simulink library "sm_boom_lift_crawler_lib_actuators"  (R2026a)
settings: Solver=ode23t
undefined symbols (not defined in the file): actuators, BasketR, cylinders, Extend, Jib, LevelM, LevelS, Lift, lines, OutFL, OutFR, OutRL, OutRR, Tilt, TrackL, TrackR, Turret, valves
libraries: SimscapeFluids_lib x92, fl_lib x67, sm_boom_lift_crawler_lib x24, nesl_utility x13, Custom_Valves x2
(part 1 of 5)
Description:
  | Boom Lift Crawler Hydraulics (Library)
  | 
  | Copyright 2020-2026 The MathWorks, Inc.
settings Model: Creator=smiller  LastModifiedBy=smiller

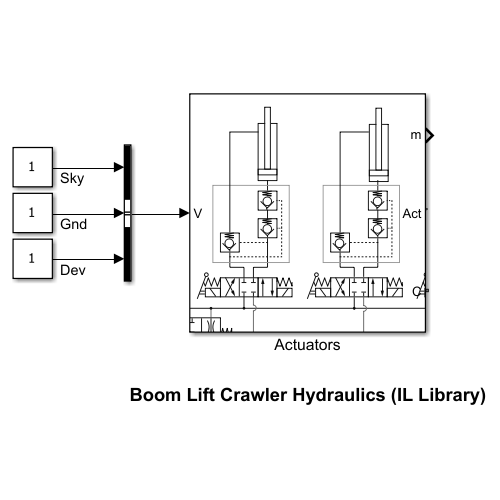
[thumbnail: Simulink's stored preview of the top-level diagram]
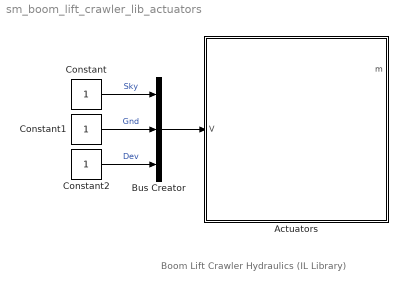
== system sm_boom_lift_crawler_lib_actuators ==
  note: Boom Lift Crawler Hydraulics (IL Library)
  Actuators : Subsystem  VariantControl=Actuators_CVs
      mask Display: image('sh001_trim_2act.svg');
  Bus Creator : BusCreator  Inputs=3
  Constant : Constant
  Constant1 : Constant
  Constant2 : Constant
  wires:
  Constant/1 -> Bus Creator/1  "Sky"
  Constant1/1 -> Bus Creator/2  "Gnd"
  Constant2/1 -> Bus Creator/3  "Dev"
  Bus Creator/1 -> Actuators/1(V)

== system sm_boom_lift_crawler_lib_actuators/Actuators ==
  In Bus Element : Inport  PortName=V  Element=Sky
  In Bus Element1 : Inport  PortName=V  Element=Gnd
  In Bus Element2 : Inport  PortName=V  Element=Dev
  Deviator Valves : Subsystem
      mask Display: image('sh002.svg')
  Ground Manifold : Subsystem
      mask Display: image('sh004.svg')
  Hydraulic Power Unit : Subsystem
      mask Display: image('sh003.svg')
  Sky Manifold : Subsystem
      mask Display: image('sh005.svg')
  Subsystem : Subsystem
  Act : PMIOPort  Side=Right
  C : PMIOPort  Port=2  Side=Right
  m : Outport
  wires:
  In Bus Element/1 -> Sky Manifold/1(Sky)
  In Bus Element2/1 -> Deviator Valves/1(Dev)
  In Bus Element1/1 -> Ground Manifold/1(Gnd)
  [G] -> Subsystem/2(G)
  [S] -> Subsystem/1(S)
  Subsystem/1(H) -> m/1  "Hydr"
  Ground Manifold/1(m) -> [G]
  Sky Manifold/1(m) -> [S]
  connections:
  Ground Manifold/RConn1 -- Sky Manifold/RConn1 -- Act/RConn1
  Sky Manifold/LConn2 -- Deviator Valves/RConn1
  Deviator Valves/RConn3 -- Ground Manifold/LConn3
  Deviator Valves/RConn2 -- Ground Manifold/LConn2
  Sky Manifold/LConn1 -- Ground Manifold/LConn1 -- Hydraulic Power Unit/LConn1 -- C/RConn1
  Deviator Valves/LConn1 -- Hydraulic Power Unit/LConn2
  Deviator Valves/LConn2 -- Hydraulic Power Unit/LConn3

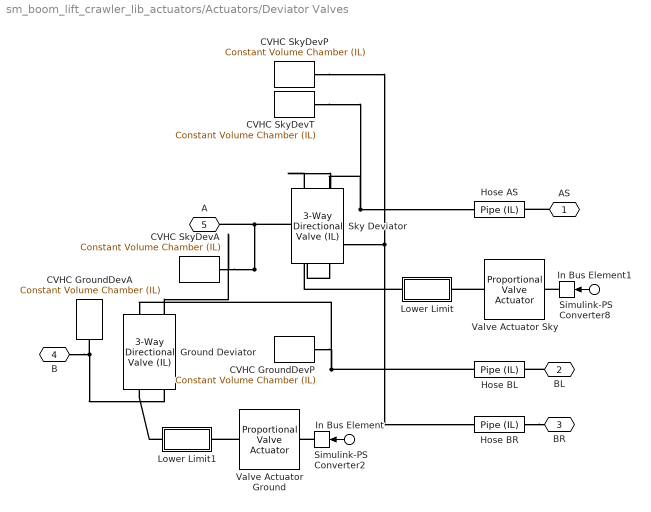
== system sm_boom_lift_crawler_lib_actuators/Actuators/Deviator Valves ==
  In Bus Element : Inport  PortName=Dev  Element=g
  In Bus Element1 : Inport  PortName=Dev  Element=s
  CVHC GroundDevA : fl_lib/Isothermal Liquid/Elements/Constant Volume Chamber (IL)  volume=1e-4 m^3  p_I_specify=off  p_I_priority=High  p_I=0 + 101325 Pa  p_I_nominal_specify=off  p_I_nominal_value=1  p_I_nominal_unit=Pa
  CVHC GroundDevP : fl_lib/Isothermal Liquid/Elements/Constant Volume Chamber (IL)  volume=1e-4 m^3  p_I_specify=off  p_I_priority=High  p_I=0 + 101325 Pa  p_I_nominal_specify=off  p_I_nominal_value=1  p_I_nominal_unit=Pa
  CVHC SkyDevA : fl_lib/Isothermal Liquid/Elements/Constant Volume Chamber (IL)  volume=1e-4 m^3  p_I_specify=off  p_I_priority=High  p_I=0 + 101325 Pa  p_I_nominal_specify=off  p_I_nominal_value=1  p_I_nominal_unit=Pa
  CVHC SkyDevP : fl_lib/Isothermal Liquid/Elements/Constant Volume Chamber (IL)  volume=1e-4 m^3  p_I_specify=off  p_I_priority=High  p_I=0 + 101325 Pa  p_I_nominal_specify=off  p_I_nominal_value=1  p_I_nominal_unit=Pa
  CVHC SkyDevT : fl_lib/Isothermal Liquid/Elements/Constant Volume Chamber (IL)  volume=1e-4 m^3  p_I_specify=off  p_I_priority=High  p_I=0 + 101325 Pa  p_I_nominal_specify=off  p_I_nominal_value=1  p_I_nominal_unit=Pa
  Ground Deviator : SimscapeFluids_lib/Isothermal Liquid/Valves & Orifices/Directional Control Valves/3-Way Directional Valve (IL)  open_orifices_pos=fluids.isothermal_liquid.valves_orifices.directional_control_valves.enum.DirectionalValveOpenOrifices3Way.PA  open_orifices_neg=fluids.isothermal_liquid.valves_orifices.directional_control_valves.enum.DirectionalValveOpenOrifices3Way.AT  area_spec=fluids.isothermal_liquid.valves_orifices.directional_control_valves.enum.directional_valve_area_spec.identical  valve_spec=fluids.isothermal_liquid.valves_orifices.directional_control_valves.enum.directional_valve_spec.linear  del_S_max=(valves.control.l.max) - 1550.0031*(valves.control.l.max)/(lines.ground.main.s.p)*(1e-12) in  area_max=lines.ground.main.s.p in^2  del_S_TLU=([-.002, 0, .002, .005, .015]) - (-0.002) m  valve_area_TLU=[1e-09, 2.0352e-07, 4.0736e-05, .00011438, .00034356] m^2  del_S_vol_flow_TLU=([-.002, 0, .002, .005, .015]) - (-0.002) m  p_diff_TLU=[-10000000, -5000000, -2000000, 2000000, 5000000, 10000000] Pa  vol_flow_TLU=[-1e-07, -7.0711e-08, -4.4721e-08, 4.4721e-08, 7.0711e-08, 1e-07; -2.0352e-05, -1.4391e-05, -9.1017e-06, 9.1017e-06, 1.4391e-05, 2.0352e-05; -.0040736, -.0028805, -.0018218, .0018218, .0028805, .0040736; -.011438, -.0080879, -.0051152, .0051152, .0080879, .011438; -.034356, -.024293, -.015364, .015364, .024293, .034356] m^3/s  area=inf m^2  area_leak=1e-12 m^2  Cd=0.7  Re_c=150  smoothing_factor=0.01  pressure_recovery=false  S_max_PA=-(0) + 0.0254*(valves.control.l.max) m  del_S_max_PA=0.005 m  area_max_PA=0.5e-4 m^2  del_S_TLU_PA=([-.002, 0, .002, .005, .015]) - (-0.002) m  valve_area_TLU_PA=[1e-09, 2.0352e-07, 4.0736e-05, .00011438, .00034356] m^2  del_S_vol_flow_TLU_PA=([-.002, 0, .002, .005, .015]) - (-0.002) m  p_diff_TLU_PA=[-10000000, -5000000, -2000000, 2000000, 5000000, 10000000] Pa  vol_flow_TLU_PA=[-1e-07, -7.0711e-08, -4.4721e-08, 4.4721e-08, 7.0711e-08, 1e-07; -2.0352e-05, -1.4391e-05, -9.1017e-06, 9.1017e-06, 1.4391e-05, 2.0352e-05; -.0040736, -.0028805, -.0018218, .0018218, .0028805, .0040736; -.011438, -.0080879, -.0051152, .0051152, .0080879, .011438; -.034356, -.024293, -.015364, .015364, .024293, .034356] m^3/s  S_max_AT=(0) - 0.0254*(valves.control.l.max) m  del_S_max_AT=0.005 m  area_max_AT=0.5e-4 m^2  del_S_TLU_AT=([-.002, 0, .002, .005, .015]) - (-0.002) m  valve_area_TLU_AT=[1e-09, 2.0352e-07, 4.0736e-05, .00011438, .00034356] m^2  del_S_vol_flow_TLU_AT=([-.002, 0, .002, .005, .015]) - (-0.002) m  p_diff_TLU_AT=[-10000000, -5000000, -2000000, 2000000, 5000000, 10000000] Pa  vol_flow_TLU_AT=[-1e-07, -7.0711e-08, -4.4721e-08, 4.4721e-08, 7.0711e-08, 1e-07; -2.0352e-05, -1.4391e-05, -9.1017e-06, 9.1017e-06, 1.4391e-05, 2.0352e-05; -.0040736, -.0028805, -.0018218, .0018218, .0028805, .0040736; -.011438, -.0080879, -.0051152, .0051152, .0080879, .011438; -.034356, -.024293, -.015364, .015364, .024293, .034356] m^3/s  S_max_PT=2.5e-3 m  del_S_max_PT=0.005 m  area_max_PT=1e-4 m^2  del_S_TLU_PT=[0, .002, .004, .007, .017] m  valve_area_TLU_PT=[1e-09, 2.0352e-07, 4.0736e-05, .00011438, .00034356] m^2  del_S_vol_flow_TLU_PT=[0, .002, .004, .007, .017] m  p_diff_TLU_PT=[.3, .5, .7] MPa  vol_flow_TLU_PT=1e-3 * [1.7e-05, 2e-05, 2.6e-05; .0035, .0045, .0053; .7, .9, 1.06; 1.96, 2.5, 3; 6, 7.7, 9.13] m^3/s
  Hose AS : SimscapeFluids_lib/Isothermal Liquid/Pipes & Fittings/Pipe (IL)  dynamic_compressibility=true  inertia=false  num_segments=1  pipe_length=lines.ground.main.l ft  cross_section_geometry=fluids.isothermal_liquid.pipes_fittings.enum.cross_section_geometry.circular  pipe_diameter=lines.ground.main.d.p in  pipe_inner_diameter=0.05 m  pipe_outer_diameter=0.1 m  pipe_width=0.1 m  pipe_height=0.1 m  pipe_major_axis=0.1 m  pipe_minor_axis=0.05 m  pipe_side=0.1 m  pipe_angle=30 deg  pipe_area=1e-4 m^2  Dh=1.12e-2 m  elevation_spec=foundation.enum.constant_variable.constant  elevation_gain=0 m  gravity_spec=foundation.enum.constant_variable.constant  g=9.81 m/s^2  pressure_loss_spec=fluids.isothermal_liquid.pipes_fittings.enum.pressure_loss_spec.haaland  mdot_nominal=[.1, 1] kg/s  p_diff_nominal=[.001, .01] MPa  mdot_threshold=1e-6 kg/s  local_pressure_loss_spec=fluids.isothermal_liquid.pipes_fittings.enum.local_loss_spec.aggregate_length  length_add=lines.ground.main.lr ft  loss_coefficient=0.1  roughness_spec=fluids.isothermal_liquid.pipes_fittings.enum.roughness_spec.custom  roughness=15e-6 m  Re_friction_TLU=[400, 1000, 1500, 3000, 4000, 6000, 10000, 20000, 40000, 60000, 100000, 100000000]  friction_factor_TLU=[.264, .112, .071, .0417, .0387, .0268, .025, .0232, .0226, .022, .0214, .0214]  Re_lam=2000  Re_tur=4000  shape_factor=64  pipe_wall_spec=fluids.isothermal_liquid.pipes_fittings.enum.wall_spec.rigid  vol_expansion_spec=fluids.isothermal_liquid.pipes_fittings.enum.vol_expansion_spec.area  area_pressure_gain=1e-6 m^2/MPa  static_pressure_TLU=[.1, 1] MPa  area_pressure_gain_TLU=[1e-05, 1.1e-05] m^2  material_behavior_spec=fluids.isothermal_liquid.pipes_fittings.enum.PipeMaterialBehavior.Linear  diameter_pressure_gain=2e-12 m/Pa  wall_thickness=0.05 m  elastic_modulus=69 GPa  stress_TLU=[276, 310] MPa  strain_TLU=[.004, .02]  stress_assert_action=simscape.enum.assert.action.none  stress_max=400 MPa  poisson_ratio=0.33  wall_time_constant=0.01 s  p0=lines.ground.main.p0 + 14.6959 psi  mdot0=0 kg/s
  Hose BL : SimscapeFluids_lib/Isothermal Liquid/Pipes & Fittings/Pipe (IL)  dynamic_compressibility=true  inertia=false  num_segments=1  pipe_length=lines.ground.main.l ft  cross_section_geometry=fluids.isothermal_liquid.pipes_fittings.enum.cross_section_geometry.circular  pipe_diameter=lines.ground.main.d.p in  pipe_inner_diameter=0.05 m  pipe_outer_diameter=0.1 m  pipe_width=0.1 m  pipe_height=0.1 m  pipe_major_axis=0.1 m  pipe_minor_axis=0.05 m  pipe_side=0.1 m  pipe_angle=30 deg  pipe_area=1e-4 m^2  Dh=1.12e-2 m  elevation_spec=foundation.enum.constant_variable.constant  elevation_gain=0 m  gravity_spec=foundation.enum.constant_variable.constant  g=9.81 m/s^2  pressure_loss_spec=fluids.isothermal_liquid.pipes_fittings.enum.pressure_loss_spec.haaland  mdot_nominal=[.1, 1] kg/s  p_diff_nominal=[.001, .01] MPa  mdot_threshold=1e-6 kg/s  local_pressure_loss_spec=fluids.isothermal_liquid.pipes_fittings.enum.local_loss_spec.aggregate_length  length_add=lines.ground.main.lr ft  loss_coefficient=0.1  roughness_spec=fluids.isothermal_liquid.pipes_fittings.enum.roughness_spec.custom  roughness=15e-6 m  Re_friction_TLU=[400, 1000, 1500, 3000, 4000, 6000, 10000, 20000, 40000, 60000, 100000, 100000000]  friction_factor_TLU=[.264, .112, .071, .0417, .0387, .0268, .025, .0232, .0226, .022, .0214, .0214]  Re_lam=2000  Re_tur=4000  shape_factor=64  pipe_wall_spec=fluids.isothermal_liquid.pipes_fittings.enum.wall_spec.rigid  vol_expansion_spec=fluids.isothermal_liquid.pipes_fittings.enum.vol_expansion_spec.area  area_pressure_gain=1e-6 m^2/MPa  static_pressure_TLU=[.1, 1] MPa  area_pressure_gain_TLU=[1e-05, 1.1e-05] m^2  material_behavior_spec=fluids.isothermal_liquid.pipes_fittings.enum.PipeMaterialBehavior.Linear  diameter_pressure_gain=2e-12 m/Pa  wall_thickness=0.05 m  elastic_modulus=69 GPa  stress_TLU=[276, 310] MPa  strain_TLU=[.004, .02]  stress_assert_action=simscape.enum.assert.action.none  stress_max=400 MPa  poisson_ratio=0.33  wall_time_constant=0.01 s  p0=lines.ground.main.p0 + 14.6959 psi  mdot0=0 kg/s
  Hose BR : SimscapeFluids_lib/Isothermal Liquid/Pipes & Fittings/Pipe (IL)  dynamic_compressibility=true  inertia=false  num_segments=1  pipe_length=lines.ground.main.l ft  cross_section_geometry=fluids.isothermal_liquid.pipes_fittings.enum.cross_section_geometry.circular  pipe_diameter=lines.ground.main.d.p in  pipe_inner_diameter=0.05 m  pipe_outer_diameter=0.1 m  pipe_width=0.1 m  pipe_height=0.1 m  pipe_major_axis=0.1 m  pipe_minor_axis=0.05 m  pipe_side=0.1 m  pipe_angle=30 deg  pipe_area=1e-4 m^2  Dh=1.12e-2 m  elevation_spec=foundation.enum.constant_variable.constant  elevation_gain=0 m  gravity_spec=foundation.enum.constant_variable.constant  g=9.81 m/s^2  pressure_loss_spec=fluids.isothermal_liquid.pipes_fittings.enum.pressure_loss_spec.haaland  mdot_nominal=[.1, 1] kg/s  p_diff_nominal=[.001, .01] MPa  mdot_threshold=1e-6 kg/s  local_pressure_loss_spec=fluids.isothermal_liquid.pipes_fittings.enum.local_loss_spec.aggregate_length  length_add=lines.ground.main.lr ft  loss_coefficient=0.1  roughness_spec=fluids.isothermal_liquid.pipes_fittings.enum.roughness_spec.custom  roughness=15e-6 m  Re_friction_TLU=[400, 1000, 1500, 3000, 4000, 6000, 10000, 20000, 40000, 60000, 100000, 100000000]  friction_factor_TLU=[.264, .112, .071, .0417, .0387, .0268, .025, .0232, .0226, .022, .0214, .0214]  Re_lam=2000  Re_tur=4000  shape_factor=64  pipe_wall_spec=fluids.isothermal_liquid.pipes_fittings.enum.wall_spec.rigid  vol_expansion_spec=fluids.isothermal_liquid.pipes_fittings.enum.vol_expansion_spec.area  area_pressure_gain=1e-6 m^2/MPa  static_pressure_TLU=[.1, 1] MPa  area_pressure_gain_TLU=[1e-05, 1.1e-05] m^2  material_behavior_spec=fluids.isothermal_liquid.pipes_fittings.enum.PipeMaterialBehavior.Linear  diameter_pressure_gain=2e-12 m/Pa  wall_thickness=0.05 m  elastic_modulus=69 GPa  stress_TLU=[276, 310] MPa  strain_TLU=[.004, .02]  stress_assert_action=simscape.enum.assert.action.none  stress_max=400 MPa  poisson_ratio=0.33  wall_time_constant=0.01 s  p0=lines.ground.main.p0 + 14.6959 psi  mdot0=0 kg/s
  Lower Limit : Subsystem
  Lower Limit1 : Subsystem
  Simulink-PS Converter2 : nesl_utility/Simulink-PS Converter  PhysicalDomain=network_engine_domain  SubClassName=ps_input  LeftPortType=input  RightPortType=output  PseudoPeriodic=off  Frequencies=[]  NoiseDistribution=none  NoiseParameters=[]  Unit=in  AffineConversion=off  FilteringAndDerivatives=provide  SimscapeFilterOrder=1  InputFilterTimeConstant=1  UdotUserProvided=0
  Simulink-PS Converter8 : nesl_utility/Simulink-PS Converter  PhysicalDomain=network_engine_domain  SubClassName=ps_input  LeftPortType=input  RightPortType=output  PseudoPeriodic=off  Frequencies=[]  NoiseDistribution=none  NoiseParameters=[]  Unit=in  AffineConversion=off  FilteringAndDerivatives=provide  SimscapeFilterOrder=1  InputFilterTimeConstant=1  UdotUserProvided=0
  Sky Deviator : SimscapeFluids_lib/Isothermal Liquid/Valves & Orifices/Directional Control Valves/3-Way Directional Valve (IL)  open_orifices_pos=fluids.isothermal_liquid.valves_orifices.directional_control_valves.enum.DirectionalValveOpenOrifices3Way.PA  open_orifices_neg=fluids.isothermal_liquid.valves_orifices.directional_control_valves.enum.DirectionalValveOpenOrifices3Way.AT  area_spec=fluids.isothermal_liquid.valves_orifices.directional_control_valves.enum.directional_valve_area_spec.identical  valve_spec=fluids.isothermal_liquid.valves_orifices.directional_control_valves.enum.directional_valve_spec.linear  del_S_max=(valves.control.l.max) - 1550.0031*(valves.control.l.max)/(lines.ground.main.s.p)*(1e-12) in  area_max=lines.ground.main.s.p in^2  del_S_TLU=([-.002, 0, .002, .005, .015]) - (-0.002) m  valve_area_TLU=[1e-09, 2.0352e-07, 4.0736e-05, .00011438, .00034356] m^2  del_S_vol_flow_TLU=([-.002, 0, .002, .005, .015]) - (-0.002) m  p_diff_TLU=[-10000000, -5000000, -2000000, 2000000, 5000000, 10000000] Pa  vol_flow_TLU=[-1e-07, -7.0711e-08, -4.4721e-08, 4.4721e-08, 7.0711e-08, 1e-07; -2.0352e-05, -1.4391e-05, -9.1017e-06, 9.1017e-06, 1.4391e-05, 2.0352e-05; -.0040736, -.0028805, -.0018218, .0018218, .0028805, .0040736; -.011438, -.0080879, -.0051152, .0051152, .0080879, .011438; -.034356, -.024293, -.015364, .015364, .024293, .034356] m^3/s  area=inf m^2  area_leak=1e-12 m^2  Cd=0.7  Re_c=150  smoothing_factor=0  pressure_recovery=false  S_max_PA=-(0) + 0.0254*(valves.control.l.max) m  del_S_max_PA=0.005 m  area_max_PA=0.5e-4 m^2  del_S_TLU_PA=([-.002, 0, .002, .005, .015]) - (-0.002) m  valve_area_TLU_PA=[1e-09, 2.0352e-07, 4.0736e-05, .00011438, .00034356] m^2  del_S_vol_flow_TLU_PA=([-.002, 0, .002, .005, .015]) - (-0.002) m  p_diff_TLU_PA=[-10000000, -5000000, -2000000, 2000000, 5000000, 10000000] Pa  vol_flow_TLU_PA=[-1e-07, -7.0711e-08, -4.4721e-08, 4.4721e-08, 7.0711e-08, 1e-07; -2.0352e-05, -1.4391e-05, -9.1017e-06, 9.1017e-06, 1.4391e-05, 2.0352e-05; -.0040736, -.0028805, -.0018218, .0018218, .0028805, .0040736; -.011438, -.0080879, -.0051152, .0051152, .0080879, .011438; -.034356, -.024293, -.015364, .015364, .024293, .034356] m^3/s  S_max_AT=(0) - 0.0254*(valves.control.l.max) m  del_S_max_AT=0.005 m  area_max_AT=0.5e-4 m^2  del_S_TLU_AT=([-.002, 0, .002, .005, .015]) - (-0.002) m  valve_area_TLU_AT=[1e-09, 2.0352e-07, 4.0736e-05, .00011438, .00034356] m^2  del_S_vol_flow_TLU_AT=([-.002, 0, .002, .005, .015]) - (-0.002) m  p_diff_TLU_AT=[-10000000, -5000000, -2000000, 2000000, 5000000, 10000000] Pa  vol_flow_TLU_AT=[-1e-07, -7.0711e-08, -4.4721e-08, 4.4721e-08, 7.0711e-08, 1e-07; -2.0352e-05, -1.4391e-05, -9.1017e-06, 9.1017e-06, 1.4391e-05, 2.0352e-05; -.0040736, -.0028805, -.0018218, .0018218, .0028805, .0040736; -.011438, -.0080879, -.0051152, .0051152, .0080879, .011438; -.034356, -.024293, -.015364, .015364, .024293, .034356] m^3/s  S_max_PT=2.5e-3 m  del_S_max_PT=0.005 m  area_max_PT=1e-4 m^2  del_S_TLU_PT=[0, .002, .004, .007, .017] m  valve_area_TLU_PT=[1e-09, 2.0352e-07, 4.0736e-05, .00011438, .00034356] m^2  del_S_vol_flow_TLU_PT=[0, .002, .004, .007, .017] m  p_diff_TLU_PT=[.3, .5, .7] MPa  vol_flow_TLU_PT=1e-3 * [1.7e-05, 2e-05, 2.6e-05; .0035, .0045, .0053; .7, .9, 1.06; 1.96, 2.5, 3; 6, 7.7, 9.13] m^3/s
  Valve Actuator Ground : SimscapeFluids_lib/Valve Actuators/Proportional Valve Actuator  gain=1 in  time_constant=0.1 s  valve_stroke=valves.control.l.max in
  Valve Actuator Sky : SimscapeFluids_lib/Valve Actuators/Proportional Valve Actuator  gain=1 in  time_constant=0.1 s  valve_stroke=valves.control.l.max in
  AS : PMIOPort  Side=Right
  BL : PMIOPort  Port=2  Side=Right
  BR : PMIOPort  Port=3  Side=Right
  B : PMIOPort  Port=4  Side=Left
  A : PMIOPort  Port=5  Side=Left
  wires:
  In Bus Element/1 -> Simulink-PS Converter2/1
  In Bus Element1/1 -> Simulink-PS Converter8/1
  connections:
  Hose BR/RConn1 -- BR/RConn1
  CVHC SkyDevT/LConn1 -- Hose AS/LConn1 -- Sky Deviator/RConn2
  Simulink-PS Converter8/RConn1 -- Valve Actuator Sky/LConn1
  Simulink-PS Converter2/RConn1 -- Valve Actuator Ground/LConn1
  AS/RConn1 -- Hose AS/RConn1
  BL/RConn1 -- Hose BL/RConn1
  Valve Actuator Sky/RConn1 -- Lower Limit/RConn1
  Valve Actuator Ground/RConn1 -- Lower Limit1/RConn1
  B/RConn1 -- Ground Deviator/LConn2 -- CVHC GroundDevA/LConn1
  Hose BL/LConn1 -- CVHC GroundDevP/LConn1 -- Ground Deviator/RConn1
  Lower Limit1/LConn1 -- Ground Deviator/LConn1
  CVHC SkyDevP/LConn1 -- Hose BR/LConn1 -- Sky Deviator/RConn1
  CVHC SkyDevA/LConn1 -- Sky Deviator/LConn2 -- A/RConn1 -- Ground Deviator/RConn2
  Lower Limit/LConn1 -- Sky Deviator/LConn1

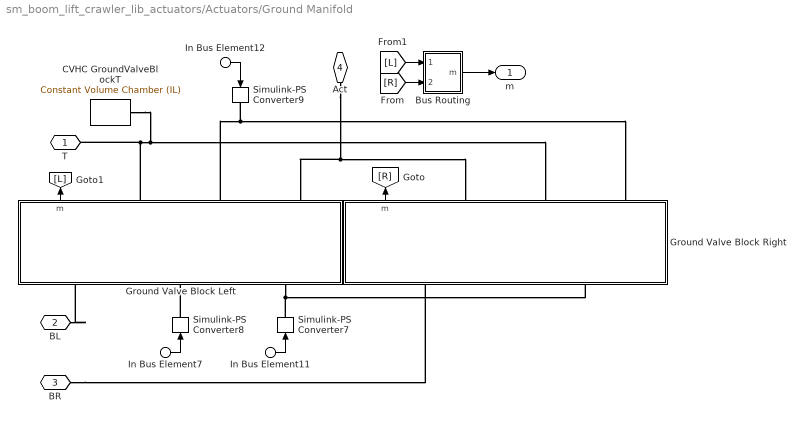
== system sm_boom_lift_crawler_lib_actuators/Actuators/Ground Manifold ==
  In Bus Element7 : Inport  PortName=Gnd  Element=Tr
  In Bus Element11 : Inport  PortName=Gnd  Element=Ou
  In Bus Element12 : Inport  PortName=Gnd  Element=Pr
  Bus Routing : Subsystem
  CVHC GroundValveBlockT : fl_lib/Isothermal Liquid/Elements/Constant Volume Chamber (IL)  volume=1e-4 m^3  p_I_specify=off  p_I_priority=High  p_I=0 + 101325 Pa  p_I_nominal_specify=off  p_I_nominal_value=1  p_I_nominal_unit=Pa
  Ground Valve Block Left : Subsystem
      mask Display: image('sh008.svg')
  Ground Valve Block Right : Subsystem
      mask Display: image('sh006.svg')
  Simulink-PS Converter7 : nesl_utility/Simulink-PS Converter  PhysicalDomain=network_engine_domain  SubClassName=ps_input  LeftPortType=input  RightPortType=output  PseudoPeriodic=off  Frequencies=[]  NoiseDistribution=none  NoiseParameters=[]  Unit=1  AffineConversion=off  FilteringAndDerivatives=provide  SimscapeFilterOrder=1  InputFilterTimeConstant=1  UdotUserProvided=0
  Simulink-PS Converter8 : nesl_utility/Simulink-PS Converter  PhysicalDomain=network_engine_domain  SubClassName=ps_input  LeftPortType=input  RightPortType=output  PseudoPeriodic=off  Frequencies=[]  NoiseDistribution=none  NoiseParameters=[]  Unit=1  AffineConversion=off  FilteringAndDerivatives=provide  SimscapeFilterOrder=1  InputFilterTimeConstant=1  UdotUserProvided=0
  Simulink-PS Converter9 : nesl_utility/Simulink-PS Converter  PhysicalDomain=network_engine_domain  SubClassName=ps_input  LeftPortType=input  RightPortType=output  PseudoPeriodic=off  Frequencies=[]  NoiseDistribution=none  NoiseParameters=[]  Unit=1  AffineConversion=off  FilteringAndDerivatives=provide  SimscapeFilterOrder=1  InputFilterTimeConstant=1  UdotUserProvided=0
  T : PMIOPort  Side=Left
  BL : PMIOPort  Port=2  Side=Left
  BR : PMIOPort  Port=3  Side=Left
  Act : PMIOPort  Port=4  Side=Right
  m : Outport
  wires:
  In Bus Element7/1 -> Simulink-PS Converter8/1
  In Bus Element11/1 -> Simulink-PS Converter7/1
  In Bus Element12/1 -> Simulink-PS Converter9/1
  Bus Routing/1(m) -> m/1
  [R] -> Bus Routing/2(m2)
  [L] -> Bus Routing/1(m1)
  Ground Valve Block Left/1(m) -> [L]
  Ground Valve Block Right/1(m) -> [R]
  connections:
  Act/RConn1 -- Ground Valve Block Left/RConn3 -- Ground Valve Block Right/RConn1
  Simulink-PS Converter8/RConn1 -- Ground Valve Block Left/LConn2
  Ground Valve Block Left/LConn3 -- Ground Valve Block Right/LConn2 -- Simulink-PS Converter7/RConn1
  Ground Valve Block Left/RConn2 -- Ground Valve Block Right/RConn3 -- Simulink-PS Converter9/RConn1
  BL/RConn1 -- Ground Valve Block Left/LConn1
  BR/RConn1 -- Ground Valve Block Right/LConn1
  Ground Valve Block Left/RConn1 -- T/RConn1 -- Ground Valve Block Right/RConn2 -- CVHC GroundValveBlockT/LConn1

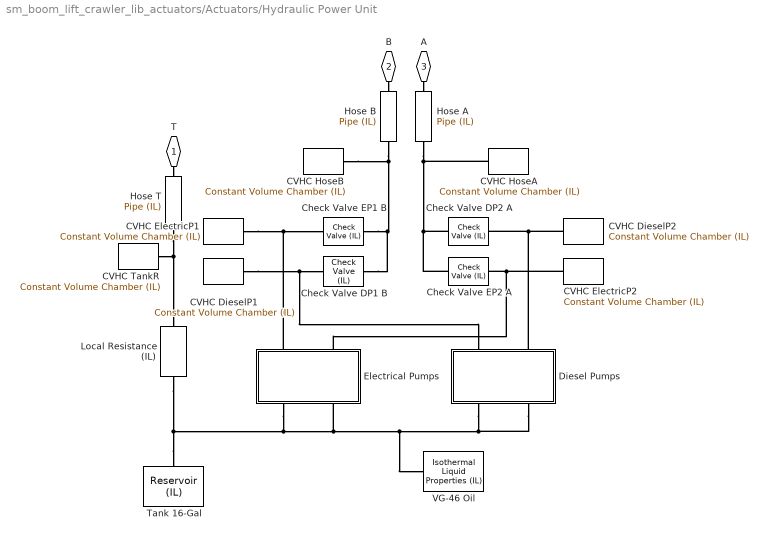
== system sm_boom_lift_crawler_lib_actuators/Actuators/Hydraulic Power Unit ==
  CVHC DieselP1 : fl_lib/Isothermal Liquid/Elements/Constant Volume Chamber (IL)  volume=1e-4 m^3  p_I_specify=off  p_I_priority=High  p_I=0 + 101325 Pa  p_I_nominal_specify=off  p_I_nominal_value=1  p_I_nominal_unit=Pa
  CVHC DieselP2 : fl_lib/Isothermal Liquid/Elements/Constant Volume Chamber (IL)  volume=1e-4 m^3  p_I_specify=off  p_I_priority=High  p_I=0 + 101325 Pa  p_I_nominal_specify=off  p_I_nominal_value=1  p_I_nominal_unit=Pa
  CVHC ElectricP1 : fl_lib/Isothermal Liquid/Elements/Constant Volume Chamber (IL)  volume=1e-4 m^3  p_I_specify=off  p_I_priority=High  p_I=0 + 101325 Pa  p_I_nominal_specify=off  p_I_nominal_value=1  p_I_nominal_unit=Pa
  CVHC ElectricP2 : fl_lib/Isothermal Liquid/Elements/Constant Volume Chamber (IL)  volume=1e-4 m^3  p_I_specify=off  p_I_priority=High  p_I=0 + 101325 Pa  p_I_nominal_specify=off  p_I_nominal_value=1  p_I_nominal_unit=Pa
  CVHC HoseA : fl_lib/Isothermal Liquid/Elements/Constant Volume Chamber (IL)  volume=1e-4 m^3  p_I_specify=off  p_I_priority=High  p_I=0 + 101325 Pa  p_I_nominal_specify=off  p_I_nominal_value=1  p_I_nominal_unit=Pa
  CVHC HoseB : fl_lib/Isothermal Liquid/Elements/Constant Volume Chamber (IL)  volume=1e-4 m^3  p_I_specify=off  p_I_priority=High  p_I=0 + 101325 Pa  p_I_nominal_specify=off  p_I_nominal_value=1  p_I_nominal_unit=Pa
  CVHC TankR : fl_lib/Isothermal Liquid/Elements/Constant Volume Chamber (IL)  volume=1e-4 m^3  p_I_specify=off  p_I_priority=High  p_I=0 + 101325 Pa  p_I_nominal_specify=off  p_I_nominal_value=1  p_I_nominal_unit=Pa
  Check Valve DP1 B : SimscapeFluids_lib/Isothermal Liquid/Valves & Orifices/Directional Control Valves/Check Valve (IL)  opening_spec=fluids.isothermal_liquid.valves_orifices.enum.PressureOpeningSpec.Linear  pressure_control_spec=fluids.isothermal_liquid.valves_orifices.enum.pressure_control_spec.dp  p_crack_differential=valves.check.p.crack psi  p_crack_gauge=0.1 MPa  press_max_differential=valves.check.p.max psi  press_max_gauge=0.2 MPa  area_max=lines.ground.main.s.p in^2  area_leak=1e-12 m^2  p_diff_TLU=[0.01 : 0.01 : 0.1] MPa  valve_area_TLU=[1e-10, 1e-05, 2e-05, 3e-05, 4e-05, 5e-05, 6e-05, 7.5e-05, 8.5e-05, .0001] m^2  vol_flow_TLU=[.000358, .045, .11, .191, .284, .39, .505, .63, .764, .905] .* 1e-3 m^3/s  area=inf m^2  Cd=0.7  Re_c=150  smoothing_factor=0  pressure_recovery=false  opening_dynamics=1  tau=0.1 s
  Check Valve DP2 A : SimscapeFluids_lib/Isothermal Liquid/Valves & Orifices/Directional Control Valves/Check Valve (IL)  opening_spec=fluids.isothermal_liquid.valves_orifices.enum.PressureOpeningSpec.Linear  pressure_control_spec=fluids.isothermal_liquid.valves_orifices.enum.pressure_control_spec.dp  p_crack_differential=valves.check.p.crack psi  p_crack_gauge=0.1 MPa  press_max_differential=valves.check.p.max psi  press_max_gauge=0.2 MPa  area_max=lines.ground.main.s.p in^2  area_leak=1e-12 m^2  p_diff_TLU=[0.01 : 0.01 : 0.1] MPa  valve_area_TLU=[1e-10, 1e-05, 2e-05, 3e-05, 4e-05, 5e-05, 6e-05, 7.5e-05, 8.5e-05, .0001] m^2  vol_flow_TLU=[.000358, .045, .11, .191, .284, .39, .505, .63, .764, .905] .* 1e-3 m^3/s  area=inf m^2  Cd=0.7  Re_c=150  smoothing_factor=0  pressure_recovery=false  opening_dynamics=1  tau=0.1 s
  Check Valve EP1 B : SimscapeFluids_lib/Isothermal Liquid/Valves & Orifices/Directional Control Valves/Check Valve (IL)  opening_spec=fluids.isothermal_liquid.valves_orifices.enum.PressureOpeningSpec.Linear  pressure_control_spec=fluids.isothermal_liquid.valves_orifices.enum.pressure_control_spec.dp  p_crack_differential=valves.check.p.crack psi  p_crack_gauge=0.1 MPa  press_max_differential=valves.check.p.max psi  press_max_gauge=0.2 MPa  area_max=lines.ground.main.s.p in^2  area_leak=1e-12 m^2  p_diff_TLU=[0.01 : 0.01 : 0.1] MPa  valve_area_TLU=[1e-10, 1e-05, 2e-05, 3e-05, 4e-05, 5e-05, 6e-05, 7.5e-05, 8.5e-05, .0001] m^2  vol_flow_TLU=[.000358, .045, .11, .191, .284, .39, .505, .63, .764, .905] .* 1e-3 m^3/s  area=inf m^2  Cd=0.7  Re_c=150  smoothing_factor=0  pressure_recovery=false  opening_dynamics=1  tau=0.1 s
  Check Valve EP2 A : SimscapeFluids_lib/Isothermal Liquid/Valves & Orifices/Directional Control Valves/Check Valve (IL)  opening_spec=fluids.isothermal_liquid.valves_orifices.enum.PressureOpeningSpec.Linear  pressure_control_spec=fluids.isothermal_liquid.valves_orifices.enum.pressure_control_spec.dp  p_crack_differential=valves.check.p.crack psi  p_crack_gauge=0.1 MPa  press_max_differential=valves.check.p.max psi  press_max_gauge=0.2 MPa  area_max=lines.ground.main.s.p in^2  area_leak=1e-12 m^2  p_diff_TLU=[0.01 : 0.01 : 0.1] MPa  valve_area_TLU=[1e-10, 1e-05, 2e-05, 3e-05, 4e-05, 5e-05, 6e-05, 7.5e-05, 8.5e-05, .0001] m^2  vol_flow_TLU=[.000358, .045, .11, .191, .284, .39, .505, .63, .764, .905] .* 1e-3 m^3/s  area=inf m^2  Cd=0.7  Re_c=150  smoothing_factor=0  pressure_recovery=false  opening_dynamics=1  tau=0.1 s
  Diesel Pumps : Subsystem
      mask Display: image('sh007.svg')
  Electrical Pumps : Subsystem
      mask Display: image('sh007.svg')
  Hose A : SimscapeFluids_lib/Isothermal Liquid/Pipes & Fittings/Pipe (IL)  dynamic_compressibility=true  inertia=false  num_segments=1  pipe_length=lines.ground.main.l ft  cross_section_geometry=fluids.isothermal_liquid.pipes_fittings.enum.cross_section_geometry.circular  pipe_diameter=lines.ground.main.d.t in  pipe_inner_diameter=0.05 m  pipe_outer_diameter=0.1 m  pipe_width=0.1 m  pipe_height=0.1 m  pipe_major_axis=0.1 m  pipe_minor_axis=0.05 m  pipe_side=0.1 m  pipe_angle=30 deg  pipe_area=1e-4 m^2  Dh=1.12e-2 m  elevation_spec=foundation.enum.constant_variable.constant  elevation_gain=0 m  gravity_spec=foundation.enum.constant_variable.constant  g=9.81 m/s^2  pressure_loss_spec=fluids.isothermal_liquid.pipes_fittings.enum.pressure_loss_spec.haaland  mdot_nominal=[.1, 1] kg/s  p_diff_nominal=[.001, .01] MPa  mdot_threshold=1e-6 kg/s  local_pressure_loss_spec=fluids.isothermal_liquid.pipes_fittings.enum.local_loss_spec.aggregate_length  length_add=lines.ground.main.lr ft  loss_coefficient=0.1  roughness_spec=fluids.isothermal_liquid.pipes_fittings.enum.roughness_spec.custom  roughness=15e-6 m  Re_friction_TLU=[400, 1000, 1500, 3000, 4000, 6000, 10000, 20000, 40000, 60000, 100000, 100000000]  friction_factor_TLU=[.264, .112, .071, .0417, .0387, .0268, .025, .0232, .0226, .022, .0214, .0214]  Re_lam=2000  Re_tur=4000  shape_factor=64  pipe_wall_spec=fluids.isothermal_liquid.pipes_fittings.enum.wall_spec.rigid  vol_expansion_spec=fluids.isothermal_liquid.pipes_fittings.enum.vol_expansion_spec.area  area_pressure_gain=1e-6 m^2/MPa  static_pressure_TLU=[.1, 1] MPa  area_pressure_gain_TLU=[1e-05, 1.1e-05] m^2  material_behavior_spec=fluids.isothermal_liquid.pipes_fittings.enum.PipeMaterialBehavior.Linear  diameter_pressure_gain=2e-12 m/Pa  wall_thickness=0.05 m  elastic_modulus=69 GPa  stress_TLU=[276, 310] MPa  strain_TLU=[.004, .02]  stress_assert_action=simscape.enum.assert.action.none  stress_max=400 MPa  poisson_ratio=0.33  wall_time_constant=0.01 s  p0=lines.ground.main.p0 + 14.6959 psi  mdot0=0 kg/s
  Hose B : SimscapeFluids_lib/Isothermal Liquid/Pipes & Fittings/Pipe (IL)  dynamic_compressibility=true  inertia=false  num_segments=1  pipe_length=lines.ground.main.l ft  cross_section_geometry=fluids.isothermal_liquid.pipes_fittings.enum.cross_section_geometry.circular  pipe_diameter=lines.ground.main.d.t in  pipe_inner_diameter=0.05 m  pipe_outer_diameter=0.1 m  pipe_width=0.1 m  pipe_height=0.1 m  pipe_major_axis=0.1 m  pipe_minor_axis=0.05 m  pipe_side=0.1 m  pipe_angle=30 deg  pipe_area=1e-4 m^2  Dh=1.12e-2 m  elevation_spec=foundation.enum.constant_variable.constant  elevation_gain=0 m  gravity_spec=foundation.enum.constant_variable.constant  g=9.81 m/s^2  pressure_loss_spec=fluids.isothermal_liquid.pipes_fittings.enum.pressure_loss_spec.haaland  mdot_nominal=[.1, 1] kg/s  p_diff_nominal=[.001, .01] MPa  mdot_threshold=1e-6 kg/s  local_pressure_loss_spec=fluids.isothermal_liquid.pipes_fittings.enum.local_loss_spec.aggregate_length  length_add=lines.ground.main.lr ft  loss_coefficient=0.1  roughness_spec=fluids.isothermal_liquid.pipes_fittings.enum.roughness_spec.custom  roughness=15e-6 m  Re_friction_TLU=[400, 1000, 1500, 3000, 4000, 6000, 10000, 20000, 40000, 60000, 100000, 100000000]  friction_factor_TLU=[.264, .112, .071, .0417, .0387, .0268, .025, .0232, .0226, .022, .0214, .0214]  Re_lam=2000  Re_tur=4000  shape_factor=64  pipe_wall_spec=fluids.isothermal_liquid.pipes_fittings.enum.wall_spec.rigid  vol_expansion_spec=fluids.isothermal_liquid.pipes_fittings.enum.vol_expansion_spec.area  area_pressure_gain=1e-6 m^2/MPa  static_pressure_TLU=[.1, 1] MPa  area_pressure_gain_TLU=[1e-05, 1.1e-05] m^2  material_behavior_spec=fluids.isothermal_liquid.pipes_fittings.enum.PipeMaterialBehavior.Linear  diameter_pressure_gain=2e-12 m/Pa  wall_thickness=0.05 m  elastic_modulus=69 GPa  stress_TLU=[276, 310] MPa  strain_TLU=[.004, .02]  stress_assert_action=simscape.enum.assert.action.none  stress_max=400 MPa  poisson_ratio=0.33  wall_time_constant=0.01 s  p0=lines.ground.main.p0 + 14.6959 psi  mdot0=0 kg/s
  Hose T : SimscapeFluids_lib/Isothermal Liquid/Pipes & Fittings/Pipe (IL)  dynamic_compressibility=true  inertia=false  num_segments=1  pipe_length=lines.ground.main.l ft  cross_section_geometry=fluids.isothermal_liquid.pipes_fittings.enum.cross_section_geometry.circular  pipe_diameter=lines.ground.main.d.t in  pipe_inner_diameter=0.05 m  pipe_outer_diameter=0.1 m  pipe_width=0.1 m  pipe_height=0.1 m  pipe_major_axis=0.1 m  pipe_minor_axis=0.05 m  pipe_side=0.1 m  pipe_angle=30 deg  pipe_area=1e-4 m^2  Dh=1.12e-2 m  elevation_spec=foundation.enum.constant_variable.constant  elevation_gain=0 m  gravity_spec=foundation.enum.constant_variable.constant  g=9.81 m/s^2  pressure_loss_spec=fluids.isothermal_liquid.pipes_fittings.enum.pressure_loss_spec.haaland  mdot_nominal=[.1, 1] kg/s  p_diff_nominal=[.001, .01] MPa  mdot_threshold=1e-6 kg/s  local_pressure_loss_spec=fluids.isothermal_liquid.pipes_fittings.enum.local_loss_spec.aggregate_length  length_add=lines.ground.main.lr ft  loss_coefficient=0.1  roughness_spec=fluids.isothermal_liquid.pipes_fittings.enum.roughness_spec.custom  roughness=15e-6 m  Re_friction_TLU=[400, 1000, 1500, 3000, 4000, 6000, 10000, 20000, 40000, 60000, 100000, 100000000]  friction_factor_TLU=[.264, .112, .071, .0417, .0387, .0268, .025, .0232, .0226, .022, .0214, .0214]  Re_lam=2000  Re_tur=4000  shape_factor=64  pipe_wall_spec=fluids.isothermal_liquid.pipes_fittings.enum.wall_spec.rigid  vol_expansion_spec=fluids.isothermal_liquid.pipes_fittings.enum.vol_expansion_spec.area  area_pressure_gain=1e-6 m^2/MPa  static_pressure_TLU=[.1, 1] MPa  area_pressure_gain_TLU=[1e-05, 1.1e-05] m^2  material_behavior_spec=fluids.isothermal_liquid.pipes_fittings.enum.PipeMaterialBehavior.Linear  diameter_pressure_gain=2e-12 m/Pa  wall_thickness=0.05 m  elastic_modulus=69 GPa  stress_TLU=[276, 310] MPa  strain_TLU=[.004, .02]  stress_assert_action=simscape.enum.assert.action.none  stress_max=400 MPa  poisson_ratio=0.33  wall_time_constant=0.01 s  p0=lines.ground.main.p0 + 14.6959 psi  mdot0=0 kg/s
  Local Resistance (IL) : SimscapeFluids_lib/Isothermal Liquid/Pipes & Fittings/Local Resistance (IL)  resistance_loss_spec=fluids.isothermal_liquid.pipes_fittings.enum.resistance_loss_spec.constant  loss_coeff_AB=1  loss_coeff_BA=1  Re_TLU=[-500, -200, -100, -50, -40, -30, -20, -10, 10, 20, 30, 40, 50, 100, 200, 500, 1000, 2000]  loss_coeff_TLU=[.65, .75, .9, 1.15, 1.35, 1.65, 2.3, 3.1, 4, 2.7, 1.8, 1.46, 1.3, .9, .65, .42, .3, .2]  flow_area=pi*(lines.ground.main.d.t)^2/4 (in)^2  Re_c=15
  "Tank 16-Gal " : fl_lib/Isothermal Liquid/Elements/Reservoir (IL)  pressure_input=false  pressure_spec=2  reservoir_pressure=0 + 14.6959 psi
  VG-46 Oil : fl_lib/Isothermal Liquid/Utilities/Isothermal Liquid Properties (IL)  rho_L_atm=867.346 kg/m^3  bulk_modulus_model=foundation.enum.bulk_modulus_model.const  beta_gain=6  beta_L_atm=1.48150e+09 Pa  nu_atm=(45.7333)*(1) cSt  p_atm=0.101325 MPa  p_min=1 Pa  properties_range_check=simscape.enum.assert.action.error  air_fraction=ratio_dissolved_air  polytropic_index=1.4  rho_g_atm=1.225 kg/m^3  air_dissolution_model=simscape.enum.onoff.off  p_crit=3 MPa
  T : PMIOPort  Side=Left
  B : PMIOPort  Port=2  Side=Left
  A : PMIOPort  Port=3  Side=Left
  connections:
  B/RConn1 -- Hose B/RConn1
  A/RConn1 -- Hose A/RConn1
  Hose T/RConn1 -- Local Resistance (IL)/LConn1 -- CVHC TankR/LConn1
  T/RConn1 -- Hose T/LConn1
  CVHC DieselP1/LConn1 -- Check Valve DP1 B/LConn1 -- Diesel Pumps/RConn1
  Diesel Pumps/RConn2 -- CVHC DieselP2/LConn1 -- Check Valve DP2 A/LConn1
  Electrical Pumps/LConn2 -- CVHC ElectricP2/LConn1 -- Check Valve EP2 A/LConn1
  Electrical Pumps/LConn1 -- CVHC ElectricP1/LConn1 -- Check Valve EP1 B/LConn1
  Check Valve EP1 B/RConn1 -- CVHC HoseB/LConn1 -- Hose B/LConn1 -- Check Valve DP1 B/RConn1
  Check Valve EP2 A/RConn1 -- Check Valve DP2 A/RConn1 -- CVHC HoseA/LConn1 -- Hose A/LConn1
  "Tank 16-Gal "/LConn1 -- Electrical Pumps/RConn2 -- Diesel Pumps/LConn2 -- Diesel Pumps/LConn1 -- VG-46 Oil/RConn1 -- Electrical Pumps/RConn1 -- Local Resistance (IL)/RConn1

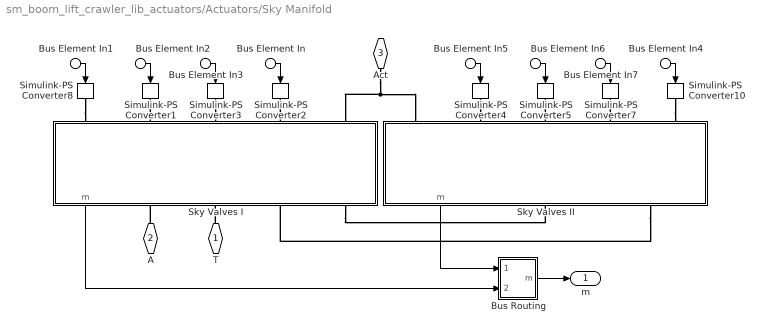
== system sm_boom_lift_crawler_lib_actuators/Actuators/Sky Manifold ==
  Bus Element In : Inport  PortName=Sky  Element=Pr
  Bus Element In1 : Inport  PortName=Sky  Element=Tu
  Bus Element In2 : Inport  PortName=Sky  Element=Li
  Bus Element In3 : Inport  PortName=Sky  Element=Ti
  Bus Element In4 : Inport  PortName=Sky  Element=BL
  Bus Element In5 : Inport  PortName=Sky  Element=Ex
  Bus Element In6 : Inport  PortName=Sky  Element=Ji
  Bus Element In7 : Inport  PortName=Sky  Element=BR
  Bus Routing : Subsystem
  Simulink-PS Converter{1..5,7..8,10} (8 alike) : nesl_utility/Simulink-PS Converter  PhysicalDomain=network_engine_domain  SubClassName=ps_input  LeftPortType=input  RightPortType=output  PseudoPeriodic=off  Frequencies=[]  NoiseDistribution=none  NoiseParameters=[]  Unit=1  AffineConversion=off  FilteringAndDerivatives=provide  SimscapeFilterOrder=1  InputFilterTimeConstant=1  UdotUserProvided=0
  Sky Valves I : Subsystem
      mask Display: image('sh011.svg')
  Sky Valves II : Subsystem
      mask Display: image('sh012.svg')
  T : PMIOPort  Side=Left
  A : PMIOPort  Port=2  Side=Left
  Act : PMIOPort  Port=3  Side=Right
  m : Outport
  wires:
  Bus Element In5/1 -> Simulink-PS Converter4/1
  Bus Element In1/1 -> Simulink-PS Converter8/1
  Bus Element In3/1 -> Simulink-PS Converter3/1
  Bus Element In2/1 -> Simulink-PS Converter1/1
  Bus Element In7/1 -> Simulink-PS Converter7/1
  Bus Element In6/1 -> Simulink-PS Converter5/1
  Bus Element In4/1 -> Simulink-PS Converter10/1
  Bus Element In/1 -> Simulink-PS Converter2/1
  Bus Routing/1(m) -> m/1
  Sky Valves II/1(m) -> Bus Routing/1(m1)
  Sky Valves I/1(m) -> Bus Routing/2(m2)
  connections:
  Act/RConn1 -- Sky Valves II/LConn1 -- Sky Valves I/LConn5
  Sky Valves II/RConn2 -- Sky Valves I/RConn3
  Sky Valves I/RConn4 -- Sky Valves II/RConn1
  Sky Valves I/LConn4 -- Simulink-PS Converter2/RConn1
  Sky Valves II/LConn4 -- Simulink-PS Converter7/RConn1
  Sky Valves II/LConn3 -- Simulink-PS Converter5/RConn1
  Sky Valves I/LConn2 -- Simulink-PS Converter1/RConn1
  Simulink-PS Converter4/RConn1 -- Sky Valves II/LConn2
  Simulink-PS Converter3/RConn1 -- Sky Valves I/LConn3
  Simulink-PS Converter8/RConn1 -- Sky Valves I/LConn1
  Simulink-PS Converter10/RConn1 -- Sky Valves II/LConn5
  T/RConn1 -- Sky Valves I/RConn2
  A/RConn1 -- Sky Valves I/RConn1

== system sm_boom_lift_crawler_lib_actuators/Actuators/Subsystem ==
  S : Inport
  G : Inport  Port=2
  Bus Creator : BusCreator  Inputs=14
  Bus Selector : BusSelector  OutputSignals=LevelS,LevelM,BasketR,Jib,Extend,Turret,Lift,Tilt
  Bus Selector1 : BusSelector  OutputSignals=TrackR,TrackL,OutFL,OutRL,OutFR,OutRR
  H : Outport
  wires:
  Bus Creator/1 -> H/1  "Hydraulic"
  G/1 -> Bus Selector1/1
  S/1 -> Bus Selector/1
  Bus Selector/1 -> Bus Creator/1  "<LevelS>"
  Bus Selector/2 -> Bus Creator/2  "<LevelM>"
  Bus Selector/3 -> Bus Creator/3  "<BasketR>"
  Bus Selector/4 -> Bus Creator/4  "<Jib>"
  Bus Selector/5 -> Bus Creator/5  "<Extend>"
  Bus Selector/6 -> Bus Creator/6  "<Turret>"
  Bus Selector/7 -> Bus Creator/7  "<Lift>"
  Bus Selector/8 -> Bus Creator/8  "<Tilt>"
  Bus Selector1/1 -> Bus Creator/9  "<TrackR>"
  Bus Selector1/2 -> Bus Creator/10  "<TrackL>"
  Bus Selector1/3 -> Bus Creator/11  "<OutFL>"
  Bus Selector1/4 -> Bus Creator/12  "<OutRL>"
  Bus Selector1/5 -> Bus Creator/13  "<OutFR>"
  Bus Selector1/6 -> Bus Creator/14  "<OutRR>"

== system sm_boom_lift_crawler_lib_actuators/Actuators/Deviator Valves/Lower Limit ==
  Min Spool Displacement : fl_lib/Physical Signals/Sources/PS Constant  constant=1e-9 m
  PS Add : fl_lib/Physical Signals/Functions/PS Add
  S : PMIOPort  Side=Right
  SLim : PMIOPort  Port=2  Side=Left
  connections:
  Min Spool Displacement/RConn1 -- PS Add/LConn2
  PS Add/RConn1 -- SLim/RConn1
  S/RConn1 -- PS Add/LConn1

== system sm_boom_lift_crawler_lib_actuators/Actuators/Deviator Valves/Lower Limit1 ==
  Min Spool Displacement : fl_lib/Physical Signals/Sources/PS Constant  constant=1e-9 m
  PS Add : fl_lib/Physical Signals/Functions/PS Add
  S : PMIOPort  Side=Right
  SLim : PMIOPort  Port=2  Side=Left
  connections:
  S/RConn1 -- PS Add/LConn1
  PS Add/RConn1 -- SLim/RConn1
  Min Spool Displacement/RConn1 -- PS Add/LConn2

== system sm_boom_lift_crawler_lib_actuators/Actuators/Ground Manifold/Bus Routing ==
  m1 : Inport
  m2 : Inport  Port=2
  Bus Creator : BusCreator  Inputs=6
  Bus Selector : BusSelector  OutputSignals=TrackR,TrackL,OutFL,OutRL
  Bus Selector1 : BusSelector  OutputSignals=OutFR,OutRR
  m : Outport
  wires:
  Bus Creator/1 -> m/1
  m1/1 -> Bus Selector/1
  m2/1 -> Bus Selector1/1
  Bus Selector1/1 -> Bus Creator/5  "<OutFR>"
  Bus Selector1/2 -> Bus Creator/6  "<OutRR>"
  Bus Selector/1 -> Bus Creator/1  "<TrackR>"
  Bus Selector/2 -> Bus Creator/2  "<TrackL>"
  Bus Selector/3 -> Bus Creator/3  "<OutFL>"
  Bus Selector/4 -> Bus Creator/4  "<OutRL>"

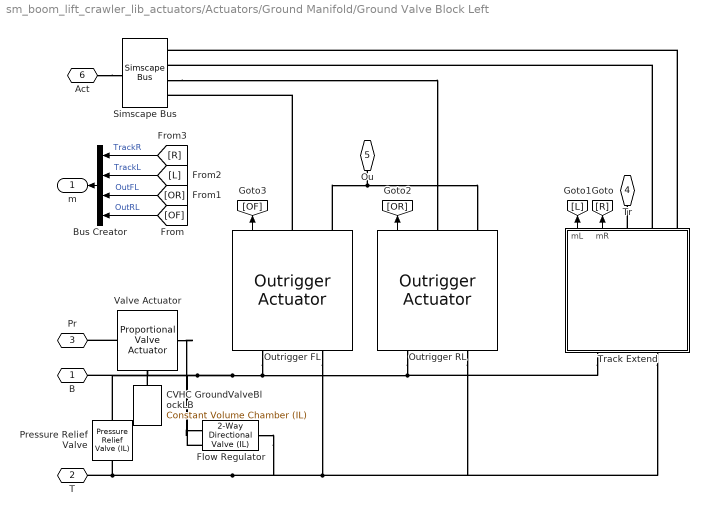
== system sm_boom_lift_crawler_lib_actuators/Actuators/Ground Manifold/Ground Valve Block Left ==
  Bus Creator : BusCreator  Inputs=4
  CVHC GroundValveBlockLB : fl_lib/Isothermal Liquid/Elements/Constant Volume Chamber (IL)  volume=1e-4 m^3  p_I_specify=off  p_I_priority=High  p_I=0 + 101325 Pa  p_I_nominal_specify=off  p_I_nominal_value=1  p_I_nominal_unit=Pa
  Flow Regulator : SimscapeFluids_lib/Isothermal Liquid/Valves & Orifices/Directional Control Valves/2-Way Directional Valve (IL)  valve_spec=1  S_max=-(0) + (valves.control.l.max) in  del_S_max=0.00064516*(-(0) + (valves.control.l.max)) - ((valves.control.l.max)/(lines.ground.main.s.t)*(1e-12) - 0.00064516*(0)) m^2/in  area_max=lines.ground.main.s.t in^2  area_leak=1e-12 m^2  del_S_TLU="[0       0.002       0.004       0.007       0.017] m"  orifice_area_TLU=[1e-09, 2.0352e-07, 4.0736e-05, .00011438, .00034356] m^2  del_S_vol_flow_TLU="[0       0.002       0.004       0.007       0.017] m"  p_diff_TLU=[-10000000, -5000000, -2000000, 2000000, 5000000, 10000000] Pa  vol_flow_TLU=[-1e-07, -7.0711e-08, -4.4721e-08, 4.4721e-08, 7.0711e-08, 1e-07; -2.0352e-05, -1.4391e-05, -9.1017e-06, 9.1017e-06, 1.4391e-05, 2.0352e-05; -.0040736, -.0028805, -.0018218, .0018218, .0028805, .0040736; -.011438, -.0080879, -.0051152, .0051152, .0080879, .011438; -.034356, -.024293, -.015364, .015364, .024293, .034356] m^3/s  Cd=0.7  Re_c=150  smoothing_factor=0  pressure_recovery=false  area=inf m^2
  Outrigger FL : sm_boom_lift_crawler_lib/Outrigger Actuator  SystemSampleTime=-1  VariantActivationTime=update diagram  EmptyChoice=off  PassThrough=off  PassThroughVariantControl=(default)  EmptyChoiceVariantControl=(default)  AllowFlexibleInterface=on  Latency=0  AutoFrameSizeCalculation=off
  Outrigger RL : sm_boom_lift_crawler_lib/Outrigger Actuator  SystemSampleTime=-1  VariantActivationTime=update diagram  EmptyChoice=off  PassThrough=off  PassThroughVariantControl=(default)  EmptyChoiceVariantControl=(default)  AllowFlexibleInterface=on  Latency=0  AutoFrameSizeCalculation=off
  Pressure Relief Valve : SimscapeFluids_lib/Isothermal Liquid/Valves & Orifices/Pressure Control Valves/Pressure Relief Valve (IL)  set_pressure_spec=foundation.enum.constant_controlled.constant  opening_spec=1  pressure_spec=fluids.isothermal_liquid.valves_orifices.enum.pressure_control_spec.dp  p_set_gauge=0.1 MPa  p_set_differential=valves.relief.p.main psi  p_range=valves.relief.dp psi  area_max=lines.ground.main.s.t in^2  area_leak=1e-12 m^2  p_diff_TLU=[30.15e5 : 15e3 : 31.35e5] Pa  p_gauge_TLU=[0.2 : 0.2 : 1.2] MPa  valve_area_TLU=[1 : 1 : 9] .* 1e-5 m^2  vol_flow_TLU=[1e-09, 3.6e-05, 8.9e-05, .00015, .00023, .00031] m^3/s  area=inf m^2  Cd=0.7  Re_c=150  smoothing_factor=0  pressure_recovery=false  opening_dynamics=1  tau=0.1 s
  Simscape Bus : SimscapeBus  HierarchyStrings=TrackR;TrackL;OutRL;OutFL
  Track Extend : Subsystem
      mask Display: image('sh010.svg')
  Valve Actuator : SimscapeFluids_lib/Valve Actuators/Proportional Valve Actuator  gain=1 in  time_constant=valves.control.tau.c s  valve_stroke=valves.control.l.max in
  B : PMIOPort  Side=Left
  T : PMIOPort  Port=2  Side=Right
  Pr : PMIOPort  Port=3  Side=Right
  Tr : PMIOPort  Port=4  Side=Left
  Ou : PMIOPort  Port=5  Side=Left
  Act : PMIOPort  Port=6  Side=Right
  m : Outport
  wires:
  Outrigger FL/1 -> [OF]
  Outrigger RL/1 -> [OR]
  Track Extend/1(mL) -> [L]
  Track Extend/2(mR) -> [R]
  [L] -> Bus Creator/2  "TrackL"
  [OR] -> Bus Creator/3  "OutFL"
  [OF] -> Bus Creator/4  "OutRL"
  [R] -> Bus Creator/1  "TrackR"
  Bus Creator/1 -> m/1
  connections:
  Track Extend/RConn3 -- Simscape Bus/LConn1
  Track Extend/RConn2 -- Simscape Bus/LConn2
  Simscape Bus/LConn3 -- Outrigger RL/RConn1
  Outrigger FL/RConn1 -- Simscape Bus/LConn4
  Act/RConn1 -- Simscape Bus/RConn1
  Outrigger FL/LConn1 -- B/RConn1 -- Pressure Relief Valve/LConn1 -- CVHC GroundValveBlockLB/LConn1 -- Flow Regulator/LConn2 -- Track Extend/LConn1 -- Outrigger RL/LConn1
  Outrigger FL/LConn2 -- Pressure Relief Valve/RConn1 -- T/RConn1 -- Flow Regulator/RConn1 -- Track Extend/LConn2 -- Outrigger RL/LConn2
  Track Extend/RConn1 -- Tr/RConn1
  Outrigger FL/RConn2 -- Ou/RConn1 -- Outrigger RL/RConn2
  Valve Actuator/RConn1 -- Flow Regulator/LConn1
  Valve Actuator/LConn1 -- Pr/RConn1

== system sm_boom_lift_crawler_lib_actuators/Actuators/Ground Manifold/Ground Valve Block Right ==
  Bus Creator : BusCreator  Inputs=2
  "CVHC GroundValveBlockRB " : fl_lib/Isothermal Liquid/Elements/Constant Volume Chamber (IL)  volume=1e-4 m^3  p_I_specify=off  p_I_priority=High  p_I=0 + 101325 Pa  p_I_nominal_specify=off  p_I_nominal_value=1  p_I_nominal_unit=Pa
  Flow Regulator : SimscapeFluids_lib/Isothermal Liquid/Valves & Orifices/Directional Control Valves/2-Way Directional Valve (IL)  valve_spec=1  S_max=-(0) + (valves.control.l.max) in  del_S_max=0.00064516*(-(0) + (valves.control.l.max)) - ((valves.control.l.max)/(lines.ground.main.s.t)*(1e-12) - 0.00064516*(0)) m^2/in  area_max=lines.ground.main.s.t in^2  area_leak=1e-12 m^2  del_S_TLU="[0       0.002       0.004       0.007       0.017] m"  orifice_area_TLU=[1e-09, 2.0352e-07, 4.0736e-05, .00011438, .00034356] m^2  del_S_vol_flow_TLU="[0       0.002       0.004       0.007       0.017] m"  p_diff_TLU=[-10000000, -5000000, -2000000, 2000000, 5000000, 10000000] Pa  vol_flow_TLU=[-1e-07, -7.0711e-08, -4.4721e-08, 4.4721e-08, 7.0711e-08, 1e-07; -2.0352e-05, -1.4391e-05, -9.1017e-06, 9.1017e-06, 1.4391e-05, 2.0352e-05; -.0040736, -.0028805, -.0018218, .0018218, .0028805, .0040736; -.011438, -.0080879, -.0051152, .0051152, .0080879, .011438; -.034356, -.024293, -.015364, .015364, .024293, .034356] m^3/s  Cd=0.7  Re_c=150  smoothing_factor=0.01  pressure_recovery=false  area=inf m^2
  Outrigger FR : sm_boom_lift_crawler_lib/Outrigger Actuator  SystemSampleTime=-1  VariantActivationTime=update diagram  EmptyChoice=off  PassThrough=off  PassThroughVariantControl=(default)  EmptyChoiceVariantControl=(default)  AllowFlexibleInterface=on  Latency=0  AutoFrameSizeCalculation=off
  Outrigger RR : sm_boom_lift_crawler_lib/Outrigger Actuator  SystemSampleTime=-1  VariantActivationTime=update diagram  EmptyChoice=off  PassThrough=off  PassThroughVariantControl=(default)  EmptyChoiceVariantControl=(default)  AllowFlexibleInterface=on  Latency=0  AutoFrameSizeCalculation=off
  Pressure Relief Valve : SimscapeFluids_lib/Isothermal Liquid/Valves & Orifices/Pressure Control Valves/Pressure Relief Valve (IL)  set_pressure_spec=foundation.enum.constant_controlled.constant  opening_spec=1  pressure_spec=fluids.isothermal_liquid.valves_orifices.enum.pressure_control_spec.dp  p_set_gauge=0.1 MPa  p_set_differential=valves.relief.p.main psi  p_range=valves.relief.dp psi  area_max=lines.ground.main.s.t in^2  area_leak=1e-12 m^2  p_diff_TLU=[30.15e5 : 15e3 : 31.35e5] Pa  p_gauge_TLU=[0.2 : 0.2 : 1.2] MPa  valve_area_TLU=[1 : 1 : 9] .* 1e-5 m^2  vol_flow_TLU=[1e-09, 3.6e-05, 8.9e-05, .00015, .00023, .00031] m^3/s  area=inf m^2  Cd=0.7  Re_c=150  smoothing_factor=0.01  pressure_recovery=false  opening_dynamics=true  tau=0.1 s
  Simscape Bus : SimscapeBus  HierarchyStrings=OutRR;OutFR
  Valve Actuator : SimscapeFluids_lib/Valve Actuators/Proportional Valve Actuator  gain=1 in  time_constant=valves.control.tau.c s  valve_stroke=valves.control.l.max in
  Act : PMIOPort  Side=Right
  T : PMIOPort  Port=2  Side=Right
  B : PMIOPort  Port=3  Side=Left
  Pr : PMIOPort  Port=4  Side=Right
  Ou : PMIOPort  Port=5  Side=Left
  m : Outport
  wires:
  [FR] -> Bus Creator/1  "OutFR"
  Bus Creator/1 -> m/1
  [RR] -> Bus Creator/2  "OutRR"
  Outrigger FR/1 -> [FR]
  Outrigger RR/1 -> [RR]
  connections:
  Simscape Bus/LConn1 -- Outrigger RR/RConn1
  Outrigger FR/RConn1 -- Simscape Bus/LConn2
  Act/RConn1 -- Simscape Bus/RConn1
  Outrigger FR/LConn2 -- Outrigger RR/LConn2 -- Pressure Relief Valve/RConn1 -- T/RConn1 -- Flow Regulator/RConn1
  Outrigger FR/LConn1 -- B/RConn1 -- Pressure Relief Valve/LConn1 -- Flow Regulator/LConn2 -- "CVHC GroundValveBlockRB "/LConn1 -- Outrigger RR/LConn1
  Valve Actuator/RConn1 -- Flow Regulator/LConn1
  Outrigger FR/RConn2 -- Ou/RConn1 -- Outrigger RR/RConn2
  Valve Actuator/LConn1 -- Pr/RConn1
